simulink model "Controle_Nivel"  (R2013a)
settings: Solver=ode45  StartTime=0.0  StopTime=40  RelTol=1e-3
libraries: fuzblock x1, neural x1
settings Model: Creator=Nielsen  LastModifiedBy=Nielsen

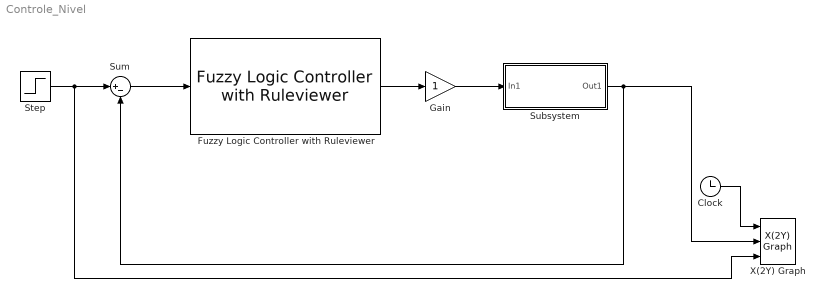
== system Controle_Nivel ==
  Clock : Clock
  Fuzzy Logic Controller with Ruleviewer : fuzblock/Fuzzy Logic  Controller  with Ruleviewer  fismatrix=tank  Ts=2
  Gain : Gain
  Step : Step  After=15  SampleTime=0
  Subsystem : Subsystem
  Sum : Sum  Inputs=|+-
  X(2Y) Graph : neural/Control Systems/X(2Y)  Graph  xmin=0  xmax=5  ymin=21  ymax=22  st=-1
  wires:
  Sum/1 -> Fuzzy Logic Controller with Ruleviewer/1
  Fuzzy Logic Controller with Ruleviewer/1 -> Gain/1
  Gain/1 -> Subsystem/1(In1)
  Clock/1 -> X(2Y) Graph/1
  Step/1 -> X(2Y) Graph/3, Sum/1
  Subsystem/1(Out1) -> X(2Y) Graph/2, Sum/2

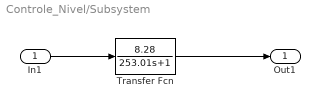
== system Controle_Nivel/Subsystem ==
  In1 : Inport
  Transfer Fcn : TransferFcn  Numerator=[8.28]  Denominator=[253.01 1]
  Out1 : Outport
  wires:
  In1/1 -> Transfer Fcn/1
  Transfer Fcn/1 -> Out1/1
